simulink model "Motor_Thermal_Model"  (R2020b)
settings: Solver=VariableStepAuto  StartTime=0.0  StopTime=6000  RelTol=1e-3
settings Model: Creator=ejrouse  LastModifiedBy=ejrouse
settings DataIOCC: ReturnWorkspaceOutputs=off
settings DebuggingCC: ArithmeticOperatorsInVariantConditions=warning
settings SFSimCC: SimUseLocalCustomCode=off  CustomCodeUndefinedFunction=UseInterfaceOnly
settings RTWCC: RTWUseLocalCustomCode=off
settings CodeAppCC: StateflowObjectComments=on

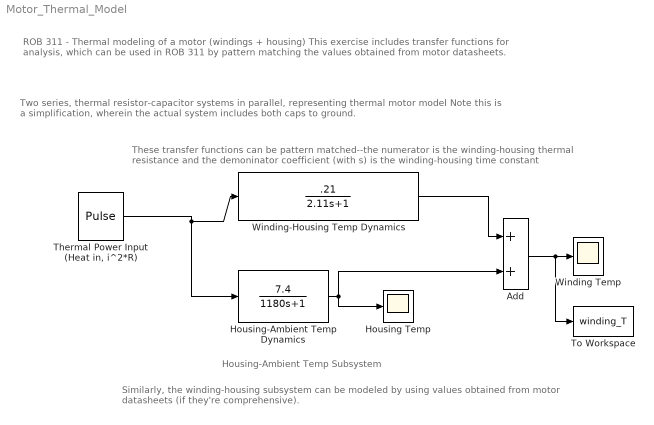
== system Motor_Thermal_Model ==
  note: ROB 311 - Thermal modeling of a motor (windings + housing)
      | This exercise includes transfer functions for analysis, which can be used in ROB 311 by pattern matching the values obtained from motor datasheets.
  note: Housing-Ambient Temp Subsystem
  note: Two series, thermal resistor-capacitor systems in parallel, representing thermal motor model
      | Note this is a simplification, wherein the actual system includes both caps to ground.
  note: These transfer functions can be pattern matched--the numerator is the winding-housing thermal resistance and the demoninator coefficient (with s) is the winding-housing time constant
  note: Similarly, the winding-housing subsystem can be modeled by using values obtained from motor datasheets (if they're comprehensive).
  Add : Sum
  Housing Temp : Scope
  Housing-Ambient Temp Dynamics : TransferFcn  Numerator=7.4  Denominator=[1180 1]
  "Thermal Power Input (Heat in, i^2*R)" : DiscretePulseGenerator  PulseType=Time based  Amplitude=(.3/.0136)^2*.102  Period=1  PulseWidth=40
  To Workspace : ToWorkspace  VariableName=winding_T  SaveFormat=Timeseries  SampleTime=-1
  Winding Temp : Scope
  Winding-Housing Temp Dynamics : TransferFcn  Numerator=[.21]  Denominator=[2.11 1]
  wires:
  Winding-Housing Temp Dynamics/1 -> Add/1
  Housing-Ambient Temp Dynamics/1 -> Add/2, Housing Temp/1
  Add/1 -> To Workspace/1, Winding Temp/1
  "Thermal Power Input (Heat in, i^2*R)"/1 -> Winding-Housing Temp Dynamics/1, Housing-Ambient Temp Dynamics/1
